simulink model "QuadCopter_3"  (R2018a)
settings: Solver=VariableStepAuto  StartTime=0.0  StopTime=t  RelTol=1e-3
values from neighbouring files (symbols this model uses):
  d = 2.4*10^-3    (= 0.0024)    [ScrValBackup.m]
  dx0 = 0    [ScrValBackup.m]
  dy0 = 0    [ScrValBackup.m]
  dz0 = 0    [ScrValBackup.m]
  g = 9.81    [ScrValBackup.m]
  Ixx = 5.9*10^-3    (= 0.0059)    [ScrValBackup.m]
  Iyy = 5.9*10^-3    (= 0.0059)    [ScrValBackup.m]
  Izz = 1.16*10^-3    (= 0.00116)    [ScrValBackup.m]
  kr = 0.1    [ScrValBackup.m]
  kt = 0.1    [ScrValBackup.m]
  l = 0.255    [ScrValBackup.m]
  m = 0.5    [ScrValBackup.m]
  p0 = 0.01    [ScrValBackup.m]
  phi0 = 5e-4    (= 0.0005)    [ScrValBackup.m]
  psi0 = 0    [ScrValBackup.m]
  q0 = -0.01    [ScrValBackup.m]
  r0 = 0.1177    [ScrValBackup.m]
  theta0 = -3e-4    (= -0.0003)    [ScrValBackup.m]
  x0 = 2    [ScrValBackup.m]
  x_coeff = A^-1*x_constr    [ScrValBackup.m]
  y0 = 3    [ScrValBackup.m]
  y_coeff = A^-1*y_constr    [ScrValBackup.m]
  z0 = 5    [ScrValBackup.m]
  z_coeff = A^-1*z_constr    [ScrValBackup.m]
libraries: simulink x5, aerolibutil x2
settings Model: Creator=giuseppe  LastModifiedBy=giuseppe
settings SolverCC: ZeroCrossAlgorithm=Adaptive
settings DebuggingCC: MaxConsecutiveZCsMsg=none

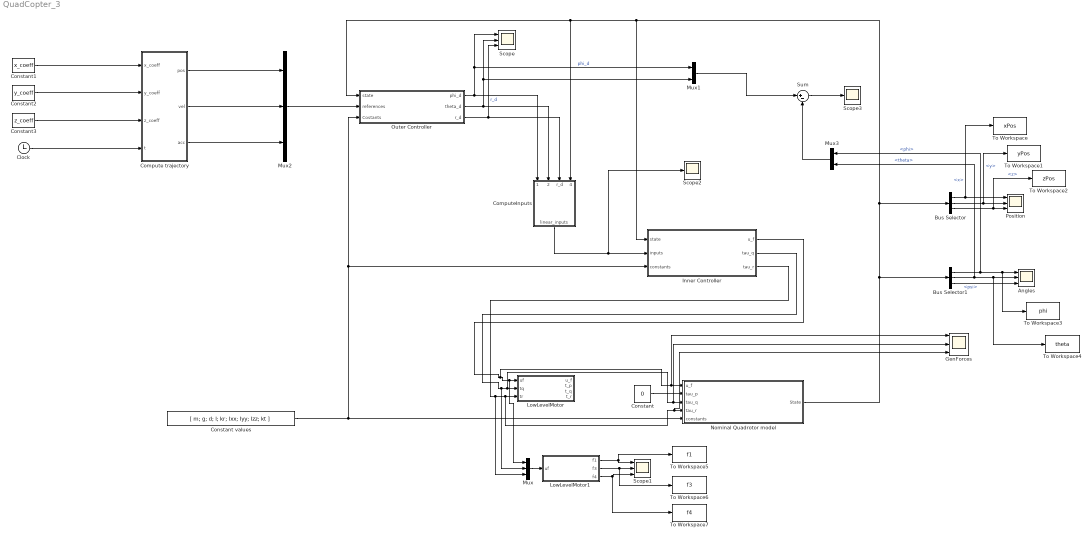
== system QuadCopter_3 ==
  Angles : Scope  NumInputPorts=3
  Bus Selector : BusSelector  OutputSignals=x,y,z
  Bus Selector1 : BusSelector  OutputSignals=phi,theta,psi
  Clock : Clock
  Compute trajectory : MATLAB Function  TreatAsAtomicUnit=on
  "ComputeInputs " : Subsystem
  Constant : Constant  Value=0
  Constant values : Constant  Value=[ m; g; d; l; kr; Ixx; Iyy; Izz; kt ]
  Constant1 : Constant  Value=x_coeff
  Constant2 : Constant  Value=y_coeff
  Constant3 : Constant  Value=z_coeff
  GenForces : Scope  NumInputPorts=3
  "Inner Controller " : Subsystem
  LowLevelMotor : Subsystem
  LowLevelMotor1 : Subsystem
  Mux : Mux  Inputs=3
  Mux1 : Mux  Inputs=2
  Mux2 : Mux  Inputs=3
  Mux3 : Mux  Inputs=2
  Nominal Quadrotor model : Subsystem
  "Outer Controller " : Subsystem
  Position : Scope  NumInputPorts=3
  Scope : Scope  NumInputPorts=3
  Scope1 : Scope  NumInputPorts=3
  Scope2 : Scope
  Scope3 : Scope
  Sum : Sum  Inputs=|+-
  To Workspace : ToWorkspace  VariableName=xPos  SaveFormat=Timeseries  SampleTime=-1
  To Workspace1 : ToWorkspace  VariableName=yPos  SaveFormat=Timeseries  SampleTime=-1
  To Workspace2 : ToWorkspace  VariableName=zPos  SaveFormat=Timeseries  SampleTime=-1
  To Workspace3 : ToWorkspace  VariableName=phi  SaveFormat=Timeseries  SampleTime=-1
  To Workspace4 : ToWorkspace  VariableName=theta  SaveFormat=Timeseries  SampleTime=-1
  To Workspace5 : ToWorkspace  VariableName=f1  SaveFormat=Timeseries  SampleTime=-1
  To Workspace6 : ToWorkspace  VariableName=f3  SaveFormat=Timeseries  SampleTime=-1
  To Workspace7 : ToWorkspace  VariableName=f4  SaveFormat=Timeseries  SampleTime=-1
  wires:
  Nominal Quadrotor model/1(State) -> "Inner Controller "/1(state), "ComputeInputs "/4(state), "Outer Controller "/1("state "), Bus Selector/1, Bus Selector1/1
  "Inner Controller "/3(tau_r) -> Mux/3, GenForces/3, Nominal Quadrotor model/4(tau_r), LowLevelMotor/3(tr)
  Constant values/1 -> "Outer Controller "/3(Costants), "Inner Controller "/3(constants), Nominal Quadrotor model/5(constants)
  "Outer Controller "/2(theta_d) -> "ComputeInputs "/2(theta_d), Mux1/2, Scope/2
  Constant3/1 -> Compute trajectory/3(z_coeff)
  "Outer Controller "/3(r_d) -> "ComputeInputs "/3(r_d), Scope/3  "r_d"
  "ComputeInputs "/1(linear_inputs) -> Scope2/1, "Inner Controller "/2(inputs)
  Constant1/1 -> Compute trajectory/1(x_coeff)
  Constant2/1 -> Compute trajectory/2(y_coeff)
  "Inner Controller "/1(u_f) -> GenForces/1, Nominal Quadrotor model/1(u_f), Mux/1, LowLevelMotor/1(uf)
  Clock/1 -> Compute trajectory/4(t)
  "Outer Controller "/1("phi_d ") -> "ComputeInputs "/1(phi_d), Mux1/1, Scope/1  "phi_d"
  Compute trajectory/3(acc) -> Mux2/3
  Compute trajectory/2(vel) -> Mux2/2
  Compute trajectory/1(pos) -> Mux2/1
  Mux2/1 -> "Outer Controller "/2(references)
  Bus Selector/1 -> To Workspace/1, Position/1  "<x>"
  Bus Selector/2 -> To Workspace1/1, Position/2  "<y>"
  Bus Selector/3 -> To Workspace2/1, Position/3  "<z>"
  Bus Selector1/1 -> Mux3/1, To Workspace3/1, Angles/1  "<phi>"
  Bus Selector1/2 -> Mux3/2, To Workspace4/1, Angles/2  "<theta>"
  Bus Selector1/3 -> Angles/3  "<psi>"
  Mux/1 -> LowLevelMotor1/1(uf)
  LowLevelMotor1/1(f1) -> Scope1/1, To Workspace5/1
  LowLevelMotor1/2(f3) -> To Workspace6/1, Scope1/2
  LowLevelMotor1/3(f4) -> To Workspace7/1, Scope1/3
  Constant/1 -> Nominal Quadrotor model/2(tau_p)
  "Inner Controller "/2(tau_q) -> Mux/2, GenForces/2, Nominal Quadrotor model/3(tau_q), LowLevelMotor/2("tq ")
  Mux3/1 -> Sum/2
  Mux1/1 -> Sum/1
  Sum/1 -> Scope3/1

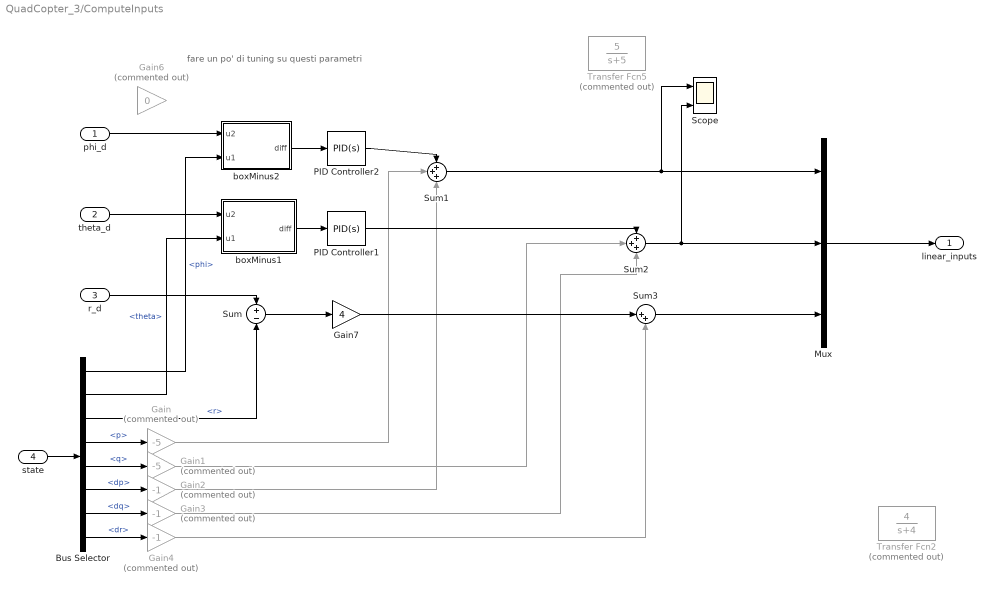
== system QuadCopter_3/ComputeInputs  ==
  note: fare un po' di tuning su questi parametri
  phi_d : Inport
  theta_d : Inport  Port=2
  r_d : Inport  Port=3
  state : Inport  Port=4
  Bus Selector : BusSelector  OutputSignals=phi,theta,r,p,q,dp,dq,dr
  Gain : Gain  Commented=on  Gain=-5
  Gain1 : Gain  Commented=on  Gain=-5
  Gain2 : Gain  Commented=on  Gain=-1
  Gain3 : Gain  Commented=on  Gain=-1
  Gain4 : Gain  Commented=on  Gain=-1
  Gain6 : Gain  Commented=on  Gain=0
  Gain7 : Gain  Gain=4
  Mux : Mux  Inputs=3
  PID Controller1 : simulink/Continuous/PID Controller  Controller=PID  TimeDomain=Continuous-time  SampleTime=-1  IntegratorMethod=Forward Euler  FilterMethod=Forward Euler  Form=Parallel  UseFilter=on  ControllerParametersSource=internal  P=100  I=10  D=30  N=100  InitialConditionSource=internal  InitialConditionForIntegrator=0  InitialConditionForFilter=0  ExternalReset=none  LimitOutput=off  UpperSaturationLimit=inf  LowerSaturationLimit=-inf  LinearizeAsGain=on  AntiWindupMode=none  Kb=1  TrackingMode=off  Kt=1  PParamMin=[]  PParamMax=[]  IParamMin=[]  IParamMax=[]  DParamMin=[]  DParamMax=[]  NParamMin=[]  NParamMax=[]  KbParamMin=[]  KbParamMax=[]  KtParamMin=[]  KtParamMax=[]  POutMin=[]  POutMax=[]  IOutMin=[]  IOutMax=[]  DOutMin=[]  DOutMax=[]  NOutMin=[]  NOutMax=[]  KbOutMin=[]  KbOutMax=[]  KtOutMin=[]  KtOutMax=[]  IntegratorOutMin=[]  IntegratorOutMax=[]  FilterOutMin=[]  FilterOutMax=[]  SumOutMin=[]  SumOutMax=[]  SumI1OutMin=[]  SumI1OutMax=[]  SumI2OutMin=[]  SumI2OutMax=[]  SumI3OutMin=[]  SumI3OutMax=[]  SumDOutMin=[]  SumDOutMax=[]  SaturationOutMin=[]  SaturationOutMax=[]  IntegratorContinuousStateAttributes=''  IntegratorStateMustResolveToSignalObject=off  IntegratorRTWStateStorageClass=Auto  FilterContinuousStateAttributes=''  FilterStateMustResolveToSignalObject=off  FilterRTWStateStorageClass=Auto  DifferentiatorICPrevScaledInput=0  DifferentiatorOutMin=[]  DifferentiatorOutMax=[]  FilterDiffOutCoefMin=[]  FilterDiffOutCoefMax=[]  SumDenOutMin=[]  SumDenOutMax=[]  SumNumOutMin=[]  SumNumOutMax=[]  ReciprocalOutMin=[]  ReciprocalOutMax=[]  DivideOutMin=[]  DivideOutMax=[]  TunerSelectOption=Transfer Function Based (PID Tuner App)
  PID Controller2 : simulink/Continuous/PID Controller  Controller=PID  TimeDomain=Continuous-time  SampleTime=-1  IntegratorMethod=Forward Euler  FilterMethod=Forward Euler  Form=Parallel  UseFilter=on  ControllerParametersSource=internal  P=100  I=10  D=30  N=100  InitialConditionSource=internal  InitialConditionForIntegrator=0  InitialConditionForFilter=0  ExternalReset=none  LimitOutput=off  UpperSaturationLimit=inf  LowerSaturationLimit=-inf  LinearizeAsGain=on  AntiWindupMode=none  Kb=1  TrackingMode=off  Kt=1  PParamMin=[]  PParamMax=[]  IParamMin=[]  IParamMax=[]  DParamMin=[]  DParamMax=[]  NParamMin=[]  NParamMax=[]  KbParamMin=[]  KbParamMax=[]  KtParamMin=[]  KtParamMax=[]  POutMin=[]  POutMax=[]  IOutMin=[]  IOutMax=[]  DOutMin=[]  DOutMax=[]  NOutMin=[]  NOutMax=[]  KbOutMin=[]  KbOutMax=[]  KtOutMin=[]  KtOutMax=[]  IntegratorOutMin=[]  IntegratorOutMax=[]  FilterOutMin=[]  FilterOutMax=[]  SumOutMin=[]  SumOutMax=[]  SumI1OutMin=[]  SumI1OutMax=[]  SumI2OutMin=[]  SumI2OutMax=[]  SumI3OutMin=[]  SumI3OutMax=[]  SumDOutMin=[]  SumDOutMax=[]  SaturationOutMin=[]  SaturationOutMax=[]  IntegratorContinuousStateAttributes=''  IntegratorStateMustResolveToSignalObject=off  IntegratorRTWStateStorageClass=Auto  FilterContinuousStateAttributes=''  FilterStateMustResolveToSignalObject=off  FilterRTWStateStorageClass=Auto  DifferentiatorICPrevScaledInput=0  DifferentiatorOutMin=[]  DifferentiatorOutMax=[]  FilterDiffOutCoefMin=[]  FilterDiffOutCoefMax=[]  SumDenOutMin=[]  SumDenOutMax=[]  SumNumOutMin=[]  SumNumOutMax=[]  ReciprocalOutMin=[]  ReciprocalOutMax=[]  DivideOutMin=[]  DivideOutMax=[]  TunerSelectOption=Transfer Function Based (PID Tuner App)
  Scope : Scope  NumInputPorts=2
  Sum : Sum  Inputs=+-
  Sum1 : Sum  Inputs=+++
  Sum2 : Sum  Inputs=+++
  Sum3 : Sum  Inputs=|++
  Transfer Fcn2 : TransferFcn  Commented=on  Numerator=[4]  Denominator=[1 4]
  Transfer Fcn5 : TransferFcn  Commented=on  Numerator=[5]  Denominator=[1 5]
  boxMinus1 : MATLAB Function  TreatAsAtomicUnit=on
  boxMinus2 : MATLAB Function  TreatAsAtomicUnit=on
  linear_inputs : Outport
  wires:
  r_d/1 -> Sum/1
  state/1 -> Bus Selector/1
  Bus Selector/1 -> boxMinus2/2(u1)  "<phi>"
  Bus Selector/2 -> boxMinus1/2(u1)  "<theta>"
  Bus Selector/3 -> Sum/2  "<r>"
  Bus Selector/4 -> Gain/1  "<p>"
  Bus Selector/5 -> Gain1/1  "<q>"
  Bus Selector/6 -> Gain2/1  "<dp>"
  Bus Selector/7 -> Gain3/1  "<dq>"
  Bus Selector/8 -> Gain4/1  "<dr>"
  boxMinus2/1(diff) -> PID Controller2/1
  Gain/1 -> Sum1/2
  Gain2/1 -> Sum1/3
  boxMinus1/1(diff) -> PID Controller1/1
  Gain1/1 -> Sum2/2
  Gain3/1 -> Sum2/3
  Sum/1 -> Gain7/1
  Gain4/1 -> Sum3/2
  Sum3/1 -> Mux/3
  Mux/1 -> linear_inputs/1
  PID Controller1/1 -> Sum2/1
  Gain7/1 -> Sum3/1
  phi_d/1 -> boxMinus2/1(u2)
  theta_d/1 -> boxMinus1/1(u2)
  PID Controller2/1 -> Sum1/1
  Sum1/1 -> Scope/1, Mux/1
  Sum2/1 -> Scope/2, Mux/2

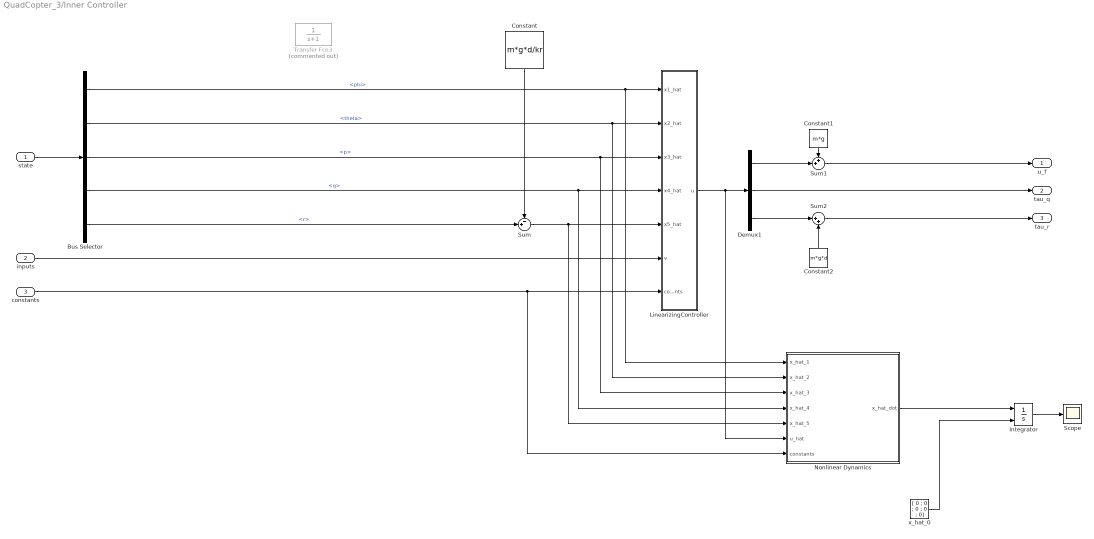
== system QuadCopter_3/Inner Controller  ==
  state : Inport
  inputs : Inport  Port=2
  constants : Inport  Port=3
  Bus Selector : BusSelector  OutputSignals=phi,theta,p,q,r
  Constant : Constant  Value=m*g*d/kr
  Constant1 : Constant  Value=m*g
  Constant2 : Constant  Value=m*g*d
  Demux1 : Demux  Outputs=3
  Integrator : Integrator  InitialConditionSource=external
  LinearizingController : MATLAB Function  TreatAsAtomicUnit=on
  "Nonlinear Dynamics " : MATLAB Function  TreatAsAtomicUnit=on
  Scope : Scope
  Sum : Sum  Inputs=-+|
  Sum1 : Sum  Inputs=++|
  Sum2 : Sum  Inputs=|++
  Transfer Fcn3 : TransferFcn  Commented=on  Denominator=[1 1]
  x_hat_0 : Constant  Value=[ 0 ; 0 ; 0 ; 0 ; 0]
  u_f : Outport
  tau_q : Outport  Port=2
  tau_r : Outport  Port=3
  wires:
  Bus Selector/3 -> "Nonlinear Dynamics "/3(x_hat_3), LinearizingController/3(x3_hat)  "<p>"
  Bus Selector/4 -> "Nonlinear Dynamics "/4(x_hat_4), LinearizingController/4(x4_hat)  "<q>"
  "Nonlinear Dynamics "/1(x_hat_dot) -> Integrator/1
  x_hat_0/1 -> Integrator/2
  Constant/1 -> Sum/1
  Sum/1 -> LinearizingController/5(x5_hat), "Nonlinear Dynamics "/5(x_hat_5)
  Demux1/3 -> Sum2/1
  Demux1/1 -> Sum1/2
  Constant1/1 -> Sum1/1
  Sum1/1 -> u_f/1
  Demux1/2 -> tau_q/1
  Constant2/1 -> Sum2/2
  Sum2/1 -> tau_r/1
  LinearizingController/1(u) -> "Nonlinear Dynamics "/6(u_hat), Demux1/1
  Integrator/1 -> Scope/1
  constants/1 -> "Nonlinear Dynamics "/7(constants), LinearizingController/7(constants)
  Bus Selector/5 -> Sum/2  "<r>"
  Bus Selector/1 -> "Nonlinear Dynamics "/1(x_hat_1), LinearizingController/1(x1_hat)  "<phi>"
  Bus Selector/2 -> "Nonlinear Dynamics "/2(x_hat_2), LinearizingController/2(x2_hat)  "<theta>"
  inputs/1 -> LinearizingController/6(v)
  state/1 -> Bus Selector/1

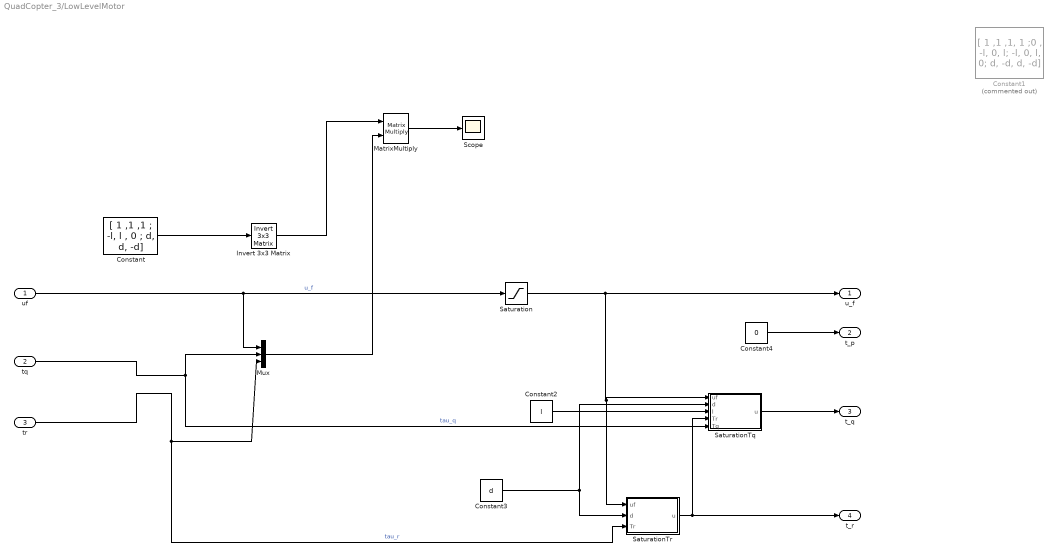
== system QuadCopter_3/LowLevelMotor ==
  uf : Inport
  "tq " : Inport  Port=2
  tr : Inport  Port=3
  Constant : Constant  Value=[ 1 ,1 ,1 ; -l, l , 0 ; d, d, -d]
  Constant1 : Constant  Commented=on  Value="[ 1 ,1 ,1, 1 ;0 , -l, 0, l;  -l, 0, l, 0; d, -d, d, -d]"
  Constant2 : Constant  Value=l
  Constant3 : Constant  Value=d
  Constant4 : Constant  Value=0
  Invert 3x3 Matrix : aerolibutil/Invert  3x3 Matrix
  MatrixMultiply : Product  Multiplication=Matrix(*)
  Mux : Mux  Inputs=3
  Saturation : Saturate  UpperLimit=15
  SaturationTq : MATLAB Function  TreatAsAtomicUnit=on
  SaturationTr : MATLAB Function  TreatAsAtomicUnit=on
  Scope : Scope
  u_f : Outport
  t_p : Outport  Port=2
  t_q : Outport  Port=3
  t_r : Outport  Port=4
  wires:
  "tq "/1 -> SaturationTq/5(Tq), Mux/2  "tau_q"
  tr/1 -> Mux/3, SaturationTr/3(Tr)  "tau_r"
  uf/1 -> Mux/1, Saturation/1  "u_f"
  Constant/1 -> Invert 3x3 Matrix/1
  Constant4/1 -> t_p/1
  Constant3/1 -> SaturationTq/2(d), SaturationTr/2(d)
  SaturationTr/1(u) -> SaturationTq/4(Tr), t_r/1
  SaturationTq/1(u) -> t_q/1
  Invert 3x3 Matrix/1 -> MatrixMultiply/1
  Saturation/1 -> SaturationTr/1(uf), SaturationTq/1(uf), u_f/1
  Mux/1 -> MatrixMultiply/2
  MatrixMultiply/1 -> Scope/1
  Constant2/1 -> SaturationTq/3(l)

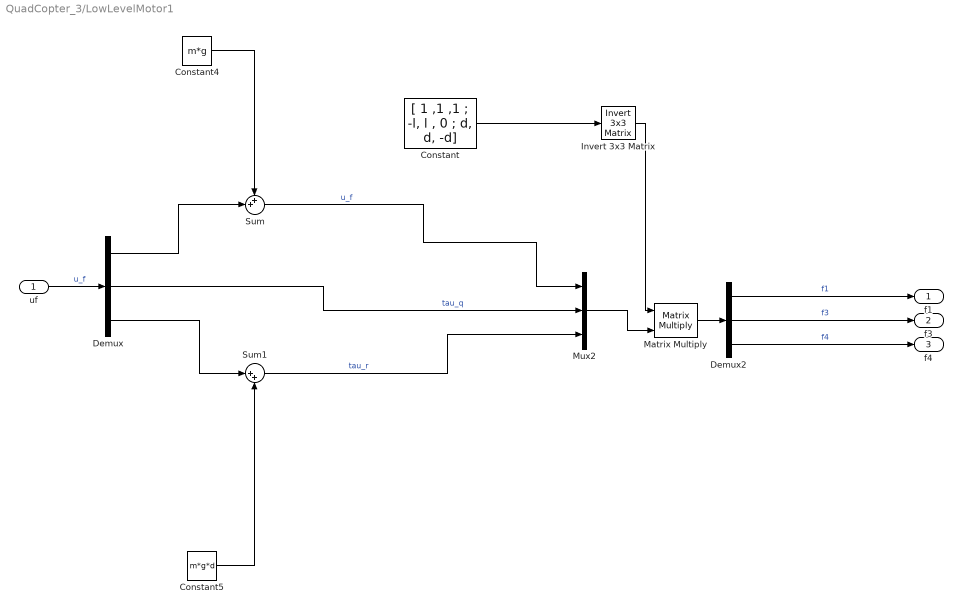
== system QuadCopter_3/LowLevelMotor1 ==
  uf : Inport
  Constant : Constant  Value=[ 1 ,1 ,1 ; -l, l , 0 ; d, d, -d]
  Constant4 : Constant  Value=m*g
  Constant5 : Constant  Value=m*g*d
  Demux : Demux  Outputs=3
  Demux2 : Demux  Outputs=3
  Invert 3x3 Matrix : aerolibutil/Invert  3x3 Matrix
  Matrix Multiply : Product  Multiplication=Matrix(*)
  Mux2 : Mux  Inputs=3
  Sum : Sum  Inputs=++|
  Sum1 : Sum  Inputs=|++
  f1 : Outport
  f3 : Outport  Port=2
  f4 : Outport  Port=3
  wires:
  Demux/2 -> Mux2/2  "tau_q"
  Invert 3x3 Matrix/1 -> Matrix Multiply/1
  Sum1/1 -> Mux2/3  "tau_r"
  Mux2/1 -> Matrix Multiply/2
  Matrix Multiply/1 -> Demux2/1
  Sum/1 -> Mux2/1  "u_f"
  Constant/1 -> Invert 3x3 Matrix/1
  uf/1 -> Demux/1  "u_f"
  Constant4/1 -> Sum/1
  Demux/1 -> Sum/2
  Demux/3 -> Sum1/1
  Constant5/1 -> Sum1/2
  Demux2/1 -> f1/1  "f1"
  Demux2/2 -> f3/1  "f3"
  Demux2/3 -> f4/1  "f4"

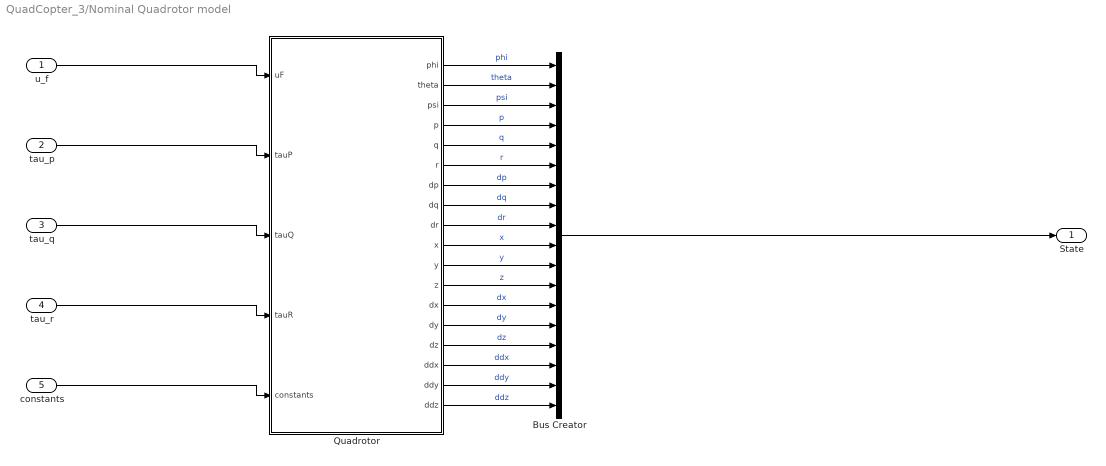
== system QuadCopter_3/Nominal Quadrotor model ==
  u_f : Inport
  tau_p : Inport  Port=2
  tau_q : Inport  Port=3
  tau_r : Inport  Port=4
  constants : Inport  Port=5
  Bus Creator : BusCreator  Inputs=18
  "Quadrotor " : Subsystem
  State : Outport
  wires:
  u_f/1 -> "Quadrotor "/1(uF)
  tau_q/1 -> "Quadrotor "/3(tauQ)
  tau_r/1 -> "Quadrotor "/4(tauR)
  constants/1 -> "Quadrotor "/5(constants)
  tau_p/1 -> "Quadrotor "/2(tauP)
  Bus Creator/1 -> State/1
  "Quadrotor "/1(phi) -> Bus Creator/1  "phi"
  "Quadrotor "/2(theta) -> Bus Creator/2  "theta"
  "Quadrotor "/3(psi) -> Bus Creator/3  "psi"
  "Quadrotor "/4(p) -> Bus Creator/4  "p"
  "Quadrotor "/5(q) -> Bus Creator/5  "q"
  "Quadrotor "/6(r) -> Bus Creator/6  "r"
  "Quadrotor "/7(dp) -> Bus Creator/7  "dp"
  "Quadrotor "/8(dq) -> Bus Creator/8  "dq"
  "Quadrotor "/9(dr) -> Bus Creator/9  "dr"
  "Quadrotor "/10(x) -> Bus Creator/10  "x"
  "Quadrotor "/11(y) -> Bus Creator/11  "y"
  "Quadrotor "/12(z) -> Bus Creator/12  "z"
  "Quadrotor "/13(dx) -> Bus Creator/13  "dx"
  "Quadrotor "/14(dy) -> Bus Creator/14  "dy"
  "Quadrotor "/15(dz) -> Bus Creator/15  "dz"
  "Quadrotor "/16(ddx) -> Bus Creator/16  "ddx"
  "Quadrotor "/17(ddy) -> Bus Creator/17  "ddy"
  "Quadrotor "/18(ddz) -> Bus Creator/18  "ddz"

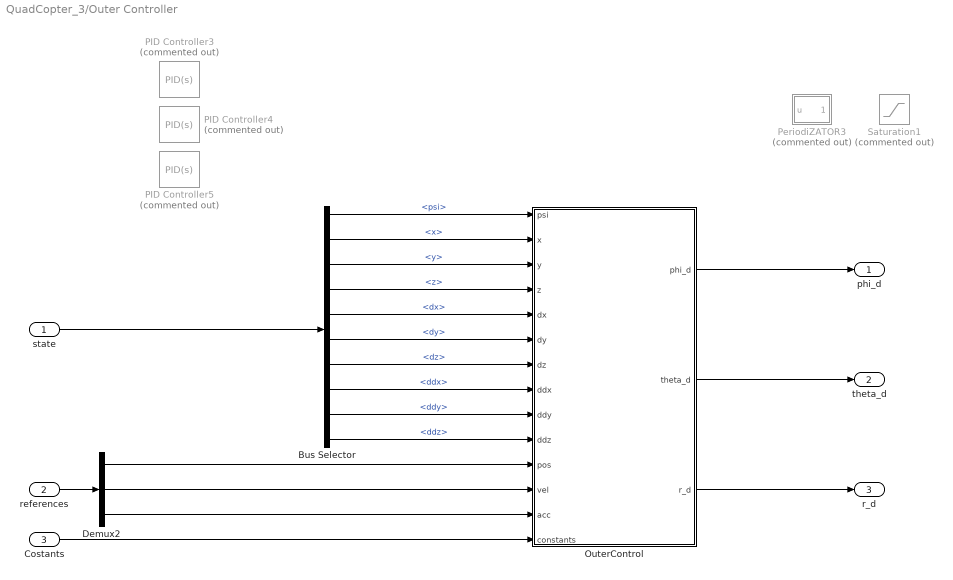
== system QuadCopter_3/Outer Controller  ==
  "state " : Inport  SampleTime=0.1
  references : Inport  Port=2
  Costants : Inport  Port=3
  Bus Selector : BusSelector  OutputSignals=psi,x,y,z,dx,dy,dz,ddx,ddy,ddz
  Demux2 : Demux  Outputs=3
  OuterControl : MATLAB Function  TreatAsAtomicUnit=on
  PID Controller3 : simulink/Continuous/PID Controller  Commented=on  Controller=PID  TimeDomain=Continuous-time  SampleTime=-1  IntegratorMethod=Forward Euler  FilterMethod=Forward Euler  Form=Parallel  UseFilter=on  ControllerParametersSource=internal  P=-3.31812549008861e-05  I=-2.04327645124417e-11  D=-11.9723513961423  N=0.0120629646409386  InitialConditionSource=internal  InitialConditionForIntegrator=0  InitialConditionForFilter=0  ExternalReset=none  LimitOutput=off  UpperSaturationLimit=inf  LowerSaturationLimit=-inf  LinearizeAsGain=on  AntiWindupMode=none  Kb=1  TrackingMode=off  Kt=1  PParamMin=[]  PParamMax=[]  IParamMin=[]  IParamMax=[]  DParamMin=[]  DParamMax=[]  NParamMin=[]  NParamMax=[]  KbParamMin=[]  KbParamMax=[]  KtParamMin=[]  KtParamMax=[]  POutMin=[]  POutMax=[]  IOutMin=[]  IOutMax=[]  DOutMin=[]  DOutMax=[]  NOutMin=[]  NOutMax=[]  KbOutMin=[]  KbOutMax=[]  KtOutMin=[]  KtOutMax=[]  IntegratorOutMin=[]  IntegratorOutMax=[]  FilterOutMin=[]  FilterOutMax=[]  SumOutMin=[]  SumOutMax=[]  SumI1OutMin=[]  SumI1OutMax=[]  SumI2OutMin=[]  SumI2OutMax=[]  SumI3OutMin=[]  SumI3OutMax=[]  SumDOutMin=[]  SumDOutMax=[]  SaturationOutMin=[]  SaturationOutMax=[]  IntegratorContinuousStateAttributes=''  IntegratorStateMustResolveToSignalObject=off  IntegratorRTWStateStorageClass=Auto  FilterContinuousStateAttributes=''  FilterStateMustResolveToSignalObject=off  FilterRTWStateStorageClass=Auto  DifferentiatorICPrevScaledInput=0  DifferentiatorOutMin=[]  DifferentiatorOutMax=[]  FilterDiffOutCoefMin=[]  FilterDiffOutCoefMax=[]  SumDenOutMin=[]  SumDenOutMax=[]  SumNumOutMin=[]  SumNumOutMax=[]  ReciprocalOutMin=[]  ReciprocalOutMax=[]  DivideOutMin=[]  DivideOutMax=[]  TunerSelectOption=Transfer Function Based (PID Tuner App)
  PID Controller4 : simulink/Continuous/PID Controller  Commented=on  Controller=PID  TimeDomain=Continuous-time  SampleTime=-1  IntegratorMethod=Forward Euler  FilterMethod=Forward Euler  Form=Parallel  UseFilter=on  ControllerParametersSource=internal  P=-3.31812549008861e-05  I=-2.04327645124417e-11  D=-11.9723513961423  N=0.0120629646409386  InitialConditionSource=internal  InitialConditionForIntegrator=0  InitialConditionForFilter=0  ExternalReset=none  LimitOutput=off  UpperSaturationLimit=inf  LowerSaturationLimit=-inf  LinearizeAsGain=on  AntiWindupMode=none  Kb=1  TrackingMode=off  Kt=1  PParamMin=[]  PParamMax=[]  IParamMin=[]  IParamMax=[]  DParamMin=[]  DParamMax=[]  NParamMin=[]  NParamMax=[]  KbParamMin=[]  KbParamMax=[]  KtParamMin=[]  KtParamMax=[]  POutMin=[]  POutMax=[]  IOutMin=[]  IOutMax=[]  DOutMin=[]  DOutMax=[]  NOutMin=[]  NOutMax=[]  KbOutMin=[]  KbOutMax=[]  KtOutMin=[]  KtOutMax=[]  IntegratorOutMin=[]  IntegratorOutMax=[]  FilterOutMin=[]  FilterOutMax=[]  SumOutMin=[]  SumOutMax=[]  SumI1OutMin=[]  SumI1OutMax=[]  SumI2OutMin=[]  SumI2OutMax=[]  SumI3OutMin=[]  SumI3OutMax=[]  SumDOutMin=[]  SumDOutMax=[]  SaturationOutMin=[]  SaturationOutMax=[]  IntegratorContinuousStateAttributes=''  IntegratorStateMustResolveToSignalObject=off  IntegratorRTWStateStorageClass=Auto  FilterContinuousStateAttributes=''  FilterStateMustResolveToSignalObject=off  FilterRTWStateStorageClass=Auto  DifferentiatorICPrevScaledInput=0  DifferentiatorOutMin=[]  DifferentiatorOutMax=[]  FilterDiffOutCoefMin=[]  FilterDiffOutCoefMax=[]  SumDenOutMin=[]  SumDenOutMax=[]  SumNumOutMin=[]  SumNumOutMax=[]  ReciprocalOutMin=[]  ReciprocalOutMax=[]  DivideOutMin=[]  DivideOutMax=[]  TunerSelectOption=Transfer Function Based (PID Tuner App)
  PID Controller5 : simulink/Continuous/PID Controller  Commented=on  Controller=PID  TimeDomain=Continuous-time  SampleTime=-1  IntegratorMethod=Forward Euler  FilterMethod=Forward Euler  Form=Parallel  UseFilter=on  ControllerParametersSource=internal  P=-3.31812549008861e-05  I=-2.04327645124417e-11  D=-11.9723513961423  N=0.0120629646409386  InitialConditionSource=internal  InitialConditionForIntegrator=0  InitialConditionForFilter=0  ExternalReset=none  LimitOutput=off  UpperSaturationLimit=inf  LowerSaturationLimit=-inf  LinearizeAsGain=on  AntiWindupMode=none  Kb=1  TrackingMode=off  Kt=1  PParamMin=[]  PParamMax=[]  IParamMin=[]  IParamMax=[]  DParamMin=[]  DParamMax=[]  NParamMin=[]  NParamMax=[]  KbParamMin=[]  KbParamMax=[]  KtParamMin=[]  KtParamMax=[]  POutMin=[]  POutMax=[]  IOutMin=[]  IOutMax=[]  DOutMin=[]  DOutMax=[]  NOutMin=[]  NOutMax=[]  KbOutMin=[]  KbOutMax=[]  KtOutMin=[]  KtOutMax=[]  IntegratorOutMin=[]  IntegratorOutMax=[]  FilterOutMin=[]  FilterOutMax=[]  SumOutMin=[]  SumOutMax=[]  SumI1OutMin=[]  SumI1OutMax=[]  SumI2OutMin=[]  SumI2OutMax=[]  SumI3OutMin=[]  SumI3OutMax=[]  SumDOutMin=[]  SumDOutMax=[]  SaturationOutMin=[]  SaturationOutMax=[]  IntegratorContinuousStateAttributes=''  IntegratorStateMustResolveToSignalObject=off  IntegratorRTWStateStorageClass=Auto  FilterContinuousStateAttributes=''  FilterStateMustResolveToSignalObject=off  FilterRTWStateStorageClass=Auto  DifferentiatorICPrevScaledInput=0  DifferentiatorOutMin=[]  DifferentiatorOutMax=[]  FilterDiffOutCoefMin=[]  FilterDiffOutCoefMax=[]  SumDenOutMin=[]  SumDenOutMax=[]  SumNumOutMin=[]  SumNumOutMax=[]  ReciprocalOutMin=[]  ReciprocalOutMax=[]  DivideOutMin=[]  DivideOutMax=[]  TunerSelectOption=Transfer Function Based (PID Tuner App)
  PeriodiZATOR3 : MATLAB Function  Commented=on  TreatAsAtomicUnit=on
  Saturation1 : Saturate  Commented=on  UpperLimit=5  LowerLimit=0
  "phi_d " : Outport
  theta_d : Outport  Port=2
  r_d : Outport  Port=3
  wires:
  Costants/1 -> OuterControl/14(constants)
  references/1 -> Demux2/1
  OuterControl/3(r_d) -> r_d/1
  OuterControl/1(phi_d) -> "phi_d "/1
  OuterControl/2(theta_d) -> theta_d/1
  "state "/1 -> Bus Selector/1
  Bus Selector/10 -> OuterControl/10(ddz)  "<ddz>"
  Bus Selector/9 -> OuterControl/9(ddy)  "<ddy>"
  Bus Selector/8 -> OuterControl/8(ddx)  "<ddx>"
  Bus Selector/7 -> OuterControl/7(dz)  "<dz>"
  Bus Selector/6 -> OuterControl/6(dy)  "<dy>"
  Bus Selector/5 -> OuterControl/5(dx)  "<dx>"
  Bus Selector/4 -> OuterControl/4(z)  "<z>"
  Bus Selector/3 -> OuterControl/3(y)  "<y>"
  Bus Selector/2 -> OuterControl/2(x)  "<x>"
  Bus Selector/1 -> OuterControl/1(psi)  "<psi>"
  Demux2/1 -> OuterControl/11(pos)
  Demux2/2 -> OuterControl/12(vel)
  Demux2/3 -> OuterControl/13(acc)

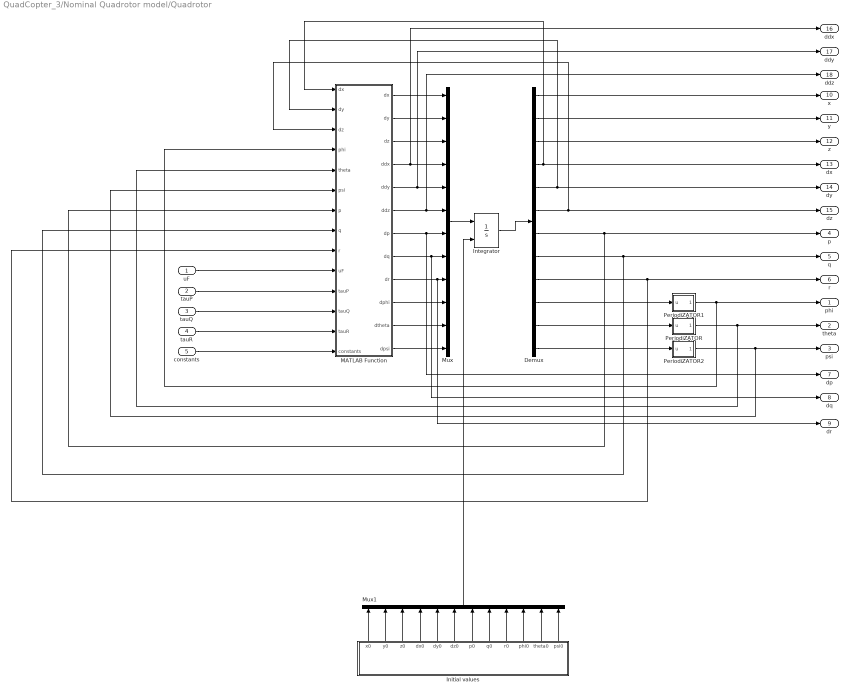
== system QuadCopter_3/Nominal Quadrotor model/Quadrotor  ==
  uF : Inport
  tauP : Inport  Port=2
  tauQ : Inport  Port=3
  tauR : Inport  Port=4
  constants : Inport  Port=5
  Demux : Demux  Outputs=12
  "Initial values " : Subsystem
  Integrator : Integrator  InitialConditionSource=external
  MATLAB Function : MATLAB Function  TreatAsAtomicUnit=on
  Mux : Mux  Inputs=12
  Mux1 : Mux  Inputs=12
  PeriodiZATOR : MATLAB Function  TreatAsAtomicUnit=on
  PeriodiZATOR1 : MATLAB Function  TreatAsAtomicUnit=on
  PeriodiZATOR2 : MATLAB Function  TreatAsAtomicUnit=on
  phi : Outport
  theta : Outport  Port=2
  psi : Outport  Port=3
  p : Outport  Port=4
  q : Outport  Port=5
  r : Outport  Port=6
  dp : Outport  Port=7
  dq : Outport  Port=8
  dr : Outport  Port=9
  x : Outport  Port=10
  y : Outport  Port=11
  z : Outport  Port=12
  dx : Outport  Port=13
  dy : Outport  Port=14
  dz : Outport  Port=15
  ddx : Outport  Port=16
  ddy : Outport  Port=17
  ddz : Outport  Port=18
  wires:
  uF/1 -> MATLAB Function/10(uF)
  tauP/1 -> MATLAB Function/11(tauP)
  tauQ/1 -> MATLAB Function/12(tauQ)
  tauR/1 -> MATLAB Function/13(tauR)
  PeriodiZATOR/1(angle) -> MATLAB Function/5(theta), theta/1
  PeriodiZATOR1/1(angle) -> MATLAB Function/4(phi), phi/1
  PeriodiZATOR2/1(angle) -> MATLAB Function/6(psi), psi/1
  constants/1 -> MATLAB Function/14(constants)
  MATLAB Function/1(dx) -> Mux/1
  MATLAB Function/2(dy) -> Mux/2
  MATLAB Function/3(dz) -> Mux/3
  MATLAB Function/4(ddx) -> ddx/1, Mux/4
  MATLAB Function/5(ddy) -> ddy/1, Mux/5
  MATLAB Function/6(ddz) -> Mux/6, ddz/1
  MATLAB Function/10(dphi) -> Mux/10
  MATLAB Function/11(dtheta) -> Mux/11
  MATLAB Function/12(dpsi) -> Mux/12
  Mux/1 -> Integrator/1
  "Initial values "/1(x0) -> Mux1/1
  "Initial values "/2(y0) -> Mux1/2
  "Initial values "/3(z0) -> Mux1/3
  "Initial values "/4(dx0) -> Mux1/4
  "Initial values "/5(dy0) -> Mux1/5
  "Initial values "/6(dz0) -> Mux1/6
  "Initial values "/7(p0) -> Mux1/7
  "Initial values "/8(q0) -> Mux1/8
  "Initial values "/9(r0) -> Mux1/9
  "Initial values "/10(phi0) -> Mux1/10
  "Initial values "/11(theta0) -> Mux1/11
  "Initial values "/12(psi0) -> Mux1/12
  Mux1/1 -> Integrator/2
  Integrator/1 -> Demux/1
  Demux/1 -> x/1
  Demux/2 -> y/1
  Demux/3 -> z/1
  Demux/5 -> dy/1, MATLAB Function/2("dy ")
  Demux/6 -> dz/1, MATLAB Function/3("dz ")
  Demux/10 -> PeriodiZATOR1/1(u)
  Demux/11 -> PeriodiZATOR/1(u)
  Demux/12 -> PeriodiZATOR2/1(u)
  Demux/9 -> MATLAB Function/9(r), r/1
  MATLAB Function/7(dp) -> Mux/7, dp/1
  MATLAB Function/8(dq) -> Mux/8, dq/1
  Demux/7 -> MATLAB Function/7(p), p/1
  Demux/8 -> MATLAB Function/8(q), q/1
  MATLAB Function/9(dr) -> dr/1, Mux/9
  Demux/4 -> dx/1, MATLAB Function/1("dx ")

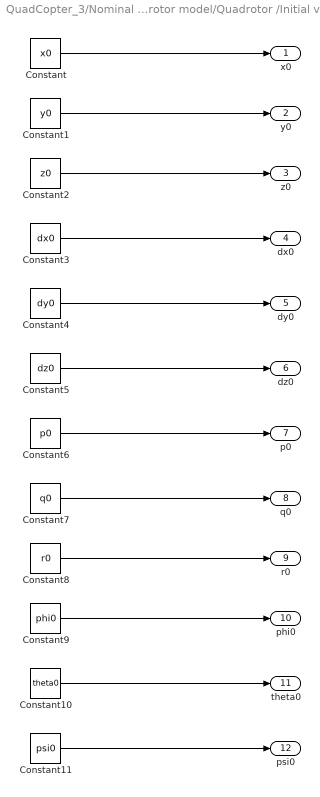
== system QuadCopter_3/Nominal Quadrotor model/Quadrotor /Initial values  ==
  Constant : Constant  Value=x0
  Constant1 : Constant  Value=y0
  Constant10 : Constant  Value=theta0
  Constant11 : Constant  Value=psi0
  Constant2 : Constant  Value=z0
  Constant3 : Constant  Value=dx0
  Constant4 : Constant  Value=dy0
  Constant5 : Constant  Value=dz0
  Constant6 : Constant  Value=p0
  Constant7 : Constant  Value=q0
  Constant8 : Constant  Value=r0
  Constant9 : Constant  Value=phi0
  x0 : Outport
  y0 : Outport  Port=2
  z0 : Outport  Port=3
  dx0 : Outport  Port=4
  dy0 : Outport  Port=5
  dz0 : Outport  Port=6
  p0 : Outport  Port=7
  q0 : Outport  Port=8
  r0 : Outport  Port=9
  phi0 : Outport  Port=10
  theta0 : Outport  Port=11
  psi0 : Outport  Port=12
  wires:
  Constant/1 -> x0/1
  Constant1/1 -> y0/1
  Constant2/1 -> z0/1
  Constant3/1 -> dx0/1
  Constant4/1 -> dy0/1
  Constant5/1 -> dz0/1
  Constant6/1 -> p0/1
  Constant7/1 -> q0/1
  Constant8/1 -> r0/1
  Constant9/1 -> phi0/1
  Constant10/1 -> theta0/1
  Constant11/1 -> psi0/1

== matlab function QuadCopter_3/Inner Controller /LinearizingController ==
  data: x1_hat input; u output; x2_hat input; x3_hat input; x4_hat input; x5_hat input; v input; constants input
function u = fcn(x1_hat,x2_hat,x3_hat,x4_hat,x5_hat, v, constants)

m= constants(1,1);
g= constants(2,1);
d= constants(3,1);
l= constants(4,1);
kr= constants(5,1);
Ixx= constants(6,1);
Iyy= constants(7,1);
Izz= constants(8,1);

alfa = zeros(3,1);

%% Non-robust feedback-linearation

alfa(1,1) = (2*Ixx*((kr*x3_hat - x4_hat*(x5_hat + (d*g*m)/kr)*(Ixx - Izz))/Ixx + (sin(x1_hat)*tan(x2_hat)*(x5_hat + (d*g*m)/kr) - x4_hat*cos(x1_hat)*tan(x2_hat))*(x3_hat + cos(x1_hat)*tan(x2_hat)*(x5_hat + (d*g*m)/kr) + x4_hat*sin(x1_hat)*tan(x2_hat)) + (sin(x1_hat)*(x5_hat + (d*g*m)/kr) - x4_hat*cos(x1_hat))*(cos(x1_hat)*(x5_hat + (d*g*m)/kr)*(tan(x2_hat)^2 + 1) + x4_hat*sin(x1_hat)*(tan(x2_hat)^2 + 1)) + (sin(x1_hat)*tan(x2_hat)*(kr*x4_hat + x3_hat*(x5_hat + (d*g*m)/kr)*(Ixx - Izz)))/Ixx + (kr*x5_hat*cos(x1_hat)*tan(x2_hat))/Izz))/l - (2*Ixx*sin(x1_hat)*tan(x2_hat)*((cos(x1_hat)*(x5_hat + (d*g*m)/kr) + x4_hat*sin(x1_hat))*(x3_hat + cos(x1_hat)*tan(x2_hat)*(x5_hat + (d*g*m)/kr) + x4_hat*sin(x1_hat)*tan(x2_hat)) + (cos(x1_hat)*(kr*x4_hat + x3_hat*(x5_hat + (d*g*m)/kr)*(Ixx - Izz)))/Ixx - (kr*x5_hat*sin(x1_hat))/Izz))/(l*cos(x1_hat)) - (kr*x5_hat*(2*Ixx*d*cos(x1_hat)^2*tan(x2_hat) - Izz*l*cos(x1_hat) + 2*Ixx*d*sin(x1_hat)^2*tan(x2_hat)))/(Izz*d*l*cos(x1_hat));
alfa(2,1) = (Ixx*((cos(x1_hat)*(x5_hat + (d*g*m)/kr) + x4_hat*sin(x1_hat))*(x3_hat + cos(x1_hat)*tan(x2_hat)*(x5_hat + (d*g*m)/kr) + x4_hat*sin(x1_hat)*tan(x2_hat)) + (cos(x1_hat)*(kr*x4_hat + x3_hat*(x5_hat + (d*g*m)/kr)*(Ixx - Izz)))/Ixx - (kr*x5_hat*sin(x1_hat))/Izz))/cos(x1_hat) + (Ixx*kr*x5_hat*sin(x1_hat))/(Izz*cos(x1_hat));
alfa(3,1) = kr*x5_hat;


beta =  [
         (2*Ixx)/l, -(2*Ixx*sin(x1_hat)*sin(x2_hat))/(l*cos(x1_hat)*cos(x2_hat)), -(2*Ixx*d*sin(x2_hat)-Izz*l*cos(x1_hat)*cos(x2_hat))/(d*l*cos(x1_hat)*cos(x2_hat));
         0,                                              Ixx/cos(x1_hat),                                                        (Ixx*sin(x1_hat))/cos(x1_hat);
         0,                                                            0,                                                                                  Izz];

%% Robust feedback linearization

% alfa(1,1) = x1_hat*((d*g*m*((2*Ixx*((d*g*m)/kr + (d*g*m*(Ixx - Izz))/(Ixx*kr)))/l + (2*kr*sin(x1_hat)*tan(x2_hat))/(l*cos(x1_hat))))/kr - (2*Ixx*d^2*g^2*m^2)/(kr^2*l)) - (sin(x1_hat)*(x5_hat + (d*g*m)/kr) - x4_hat*cos(x1_hat))*((2*Ixx*((d*g*m)/kr + (d*g*m*(Ixx - Izz))/(Ixx*kr)))/l + (2*kr*sin(x1_hat)*tan(x2_hat))/(l*cos(x1_hat))) + x2_hat*((d*g*m*((2*kr)/l - (2*Ixx*sin(x1_hat)*tan(x2_hat)*((d*g*m)/kr + (d*g*m*(Ixx - Izz))/(Ixx*kr)))/(l*cos(x1_hat))))/kr + (2*Ixx*d^2*g^2*m^2*sin(x1_hat)*tan(x2_hat))/(kr^2*l*cos(x1_hat))) - ((2*kr)/l - (2*Ixx*sin(x1_hat)*tan(x2_hat)*((d*g*m)/kr + (d*g*m*(Ixx - Izz))/(Ixx*kr)))/(l*cos(x1_hat)))*(x3_hat + cos(x1_hat)*tan(x2_hat)*(x5_hat + (d*g*m)/kr) + x4_hat*sin(x1_hat)*tan(x2_hat)) + (2*Ixx*((kr*x3_hat - x4_hat*(x5_hat + (d*g*m)/kr)*(Ixx - Izz))/Ixx + (sin(x1_hat)*tan(x2_hat)*(x5_hat + (d*g*m)/kr) - x4_hat*cos(x1_hat)*tan(x2_hat))*(x3_hat + cos(x1_hat)*tan(x2_hat)*(x5_hat + (d*g*m)/kr) + x4_hat*sin(x1_hat)*tan(x2_hat)) + (sin(x1_hat)*(x5_hat + (d*g*m)/kr) - x4_hat*cos(x1_hat))*(cos(x1_hat)*(x5_hat + (d*g*m)/kr)*(tan(x2_hat)^2 + 1) + x4_hat*sin(x1_hat)*(tan(x2_hat)^2 + 1)) + (sin(x1_hat)*tan(x2_hat)*(kr*x4_hat + x3_hat*(x5_hat + (d*g*m)/kr)*(Ixx - Izz)))/Ixx + (kr*x5_hat*cos(x1_hat)*tan(x2_hat))/Izz))/l - (2*Ixx*sin(x1_hat)*tan(x2_hat)*((cos(x1_hat)*(x5_hat + (d*g*m)/kr) + x4_hat*sin(x1_hat))*(x3_hat + cos(x1_hat)*tan(x2_hat)*(x5_hat + (d*g*m)/kr) + x4_hat*sin(x1_hat)*tan(x2_hat)) + (cos(x1_hat)*(kr*x4_hat + x3_hat*(x5_hat + (d*g*m)/kr)*(Ixx - Izz)))/Ixx - (kr*x5_hat*sin(x1_hat))/Izz))/(l*cos(x1_hat));
% alfa(2,1) = (kr*x5_hat*sin(x1_hat) - kr*x4_hat*cos(x1_hat) + d*g*m*sin(x1_hat))/cos(x1_hat) + (Ixx*((cos(x1_hat)*(kr*x4_hat + (x3_hat*(kr*x5_hat + d*g*m)*(Ixx - Izz))/kr))/Ixx + ((kr*x5_hat*cos(x1_hat) + kr*x4_hat*sin(x1_hat) + d*g*m*cos(x1_hat))*(x3_hat + x4_hat*sin(x1_hat)*tan(x2_hat) + (cos(x1_hat)*tan(x2_hat)*(kr*x5_hat + d*g*m))/kr))/kr - (kr*x5_hat*sin(x1_hat))/Izz))/cos(x1_hat) - (d*g*m*x1_hat)/cos(x1_hat) - (d*g*m*(2*Ixx - Izz)*(x3_hat + x4_hat*sin(x1_hat)*tan(x2_hat) + (cos(x1_hat)*tan(x2_hat)*(kr*x5_hat + d*g*m))/kr))/(kr*cos(x1_hat)) + (d^2*g^2*m^2*x2_hat*(Ixx - Izz))/(kr^2*cos(x1_hat));
% alfa(3,1) = 0;
% 
% beta = [
%         1, -(2*sin(x1_hat)*sin(x2_hat))/(l*cos(x1_hat)*cos(x2_hat)), -(2*Ixx*sin(x2_hat))/(Izz*l*cos(x1_hat)*cos(x2_hat));
%         0,                                            1/cos(x1_hat),                  (Ixx*sin(x1_hat))/(Izz*cos(x1_hat));
%         0,                                                        0,                                                    1];
    
u = alfa + beta*v;

== matlab function QuadCopter_3/LowLevelMotor/SaturationTr ==
  data: uf input; u output; d input; Tr input
function u = fcn(uf, d, Tr)

if abs(Tr) > d*uf
    Tr = sign(Tr)*d*uf;
end

u = Tr;

== matlab function QuadCopter_3/Inner Controller /Nonlinear Dynamics  ==
  data: x_hat_1 input; x_hat_2 input; x_hat_3 input; x_hat_4 input; x_hat_5 input; x_hat_dot output; u_hat input; constants input
function x_hat_dot = fcn(x_hat_1,x_hat_2,x_hat_3,x_hat_4,x_hat_5,u_hat,constants)

m= constants(1,1);
g= constants(2,1);
d= constants(3,1);
l= constants(4,1);
kr= constants(5,1);
Ixx= constants(6,1);
Iyy= constants(7,1);
Izz= constants(8,1);

x_hat = [x_hat_1;
        x_hat_2;
        x_hat_3;
        x_hat_4;
        x_hat_5];

f = [
    x_hat(3,1)+x_hat(4,1)*sin(x_hat(1,1))*tan(x_hat(2,1)) + ( x_hat(5,1)+ m*g*d/kr)*cos(x_hat(1,1))*tan(x_hat(2,1));
    x_hat(4,1)*cos(x_hat(1,1))- (x_hat(5,1)+ m*g*d/kr)*sin(x_hat(1,1)) ;
    1/Ixx*( -kr*x_hat(3,1)- x_hat(4,1)*(x_hat(5,1)+ m*g*d/kr)*(Izz - Ixx));
    1/Iyy*( -kr*x_hat(4,1)- x_hat(3,1)*(x_hat(5,1)+ m*g*d/kr)*(Ixx - Izz));
    1/Izz*(-kr* x_hat(5,1));    
    ];
G = [
    0 , 0 , 0;
    0,  0 , 0;
    l/(2*Ixx), 0 , -l/(2*d*Ixx)
    0,  1/Iyy  , 0 ;
    0 ,  0   ,  1/Izz;
    ];

    
x_hat_dot = f + G*u_hat;

== matlab function QuadCopter_3/LowLevelMotor/SaturationTq ==
  data: uf input; u output; d input; l input; Tr input; Tq input
function u = fcn(uf, d, l, Tr, Tq)

if abs(Tq) > (0.5*l*(uf+Tr/d))
    Tq = sign(Tq)*(0.5*l*(uf+Tr/d));
end

u = Tq;

== matlab function QuadCopter_3/ComputeInputs /boxMinus1 ==
  data: u2 input; diff output; u1 input
function diff = fcn(u2, u1)

R2 = [cos(u2) -sin(u2);
      sin(u2) cos(u2)];

R1 = [cos(-u1) -sin(-u1);
      sin(-u1) cos(-u1)];

R = R2*R1;

diff = atan2(R(2,1), R(1,1));

== matlab function QuadCopter_3/ComputeInputs /boxMinus2 ==
  data: u2 input; diff output; u1 input
function diff = fcn(u2, u1)

R2 = [cos(u2) -sin(u2);
      sin(u2) cos(u2)];

R1 = [cos(-u1) -sin(-u1);
      sin(-u1) cos(-u1)];

R = R2*R1;

diff = atan2(R(2,1), R(1,1));

== matlab function QuadCopter_3/Compute trajectory ==
  data: x_coeff input; pos output; y_coeff input; z_coeff input; t input; vel output; acc output
function [pos, vel, acc]  = fcn(x_coeff, y_coeff, z_coeff, t)

x = x_coeff(1)*t^3+x_coeff(2)*t^2+x_coeff(3)*t+x_coeff(4);
y = y_coeff(1)*t^3+y_coeff(2)*t^2+y_coeff(3)*t+y_coeff(4);
z = z_coeff(1)*t^3+z_coeff(2)*t^2+z_coeff(3)*t+z_coeff(4);

x_dot = 3*x_coeff(1)*t^2 +2*x_coeff(2)*t + x_coeff(3);
y_dot = 3*y_coeff(1)*t^2 +2*y_coeff(2)*t + y_coeff(3);
z_dot = 3*z_coeff(1)*t^2 +2*z_coeff(2)*t + z_coeff(3);

x_ddot = 6*x_coeff(1)*t+2*x_coeff(2);
y_ddot = 6*y_coeff(1)*t+2*y_coeff(2);
z_ddot = 6*z_coeff(1)*t+2*z_coeff(2);

u = zeros(3,1);

pos = [x, y, z]';
vel = [x_dot, y_dot, z_dot]';
acc = [x_ddot, y_ddot, z_ddot]';

== matlab function QuadCopter_3/Outer Controller /OuterControl ==
  data: psi input; x input; y input; z input; dx input; dy input; dz input; ddx input; ddy input; ddz input; phi_d output; pos input; vel input; acc input; theta_d output; r_d output; constants input
function [phi_d , theta_d , r_d ] = fcn(psi, x, y, z, dx, dy, dz, ddx, ddy, ddz, pos, vel, acc, constants)

m= constants(1,1);
g= constants(2,1);
d= constants(3,1);
l= constants(4,1);
kr= constants(5,1);
Ixx= constants(6,1);
Iyy= constants(7,1);
Izz= constants(8,1);
kt= constants(9,1);

xr = pos(1);
yr = pos(2);
zr = pos(3);

dxr = vel(1);
dyr = vel(2);
dzr = vel(3);

ddxr = acc(1);
ddyr = acc(2);
ddzr = acc(3);

R = [sin(psi), -cos(psi);
     cos(psi), sin(psi)];

% ux = kt/m*dx + ddxr + 0.008*(dxr -dx) + 0.03*(xr -x);
% uy = kt/m*dy + ddyr + 0.008*(dyr -dy) + 0.03*(yr -y);
% uz = kt/m*dz + ddzr + 0.5*(dzr -dz) + 0.15*(zr -z) + g;
ux = kt/m*dx + ddxr + 0.01*(dxr -dx) + 0.035*(xr -x);
uy = kt/m*dy + ddyr + 0.01*(dyr -dy) + 0.035*(yr -y);
uz = kt/m*dz + ddzr + 0.5*(dzr -dz) + 0.15*(zr -z) + g;

u = R*[ux, uy]';

r_d = uz*m*d/kr;
phi_d= u(2)/uz;
theta_d = u(1)/uz;

== matlab function QuadCopter_3/Nominal Quadrotor model/Quadrotor /MATLAB Function ==
  data: dx output; dy output; dz output; dx input; dy input; dz input; phi input; theta input; psi input; p input; q input; r input; uF input; ddx output; tauP input; tauQ input; tauR input; ddy output; ddz output; dp output; dq output; dr output; dphi output; dtheta output; dpsi output; constants input
function [dx,dy,dz,ddx,ddy,ddz,dp,dq,dr,dphi,dtheta,dpsi] = fcn(dx, dy, dz, phi, theta, psi, p, q, r, uF, tauP, tauQ, tauR, constants)

    m= constants(1,1);
    g= constants(2,1);
    d= constants(3,1);
    l= constants(4,1);
    kr= constants(5,1);
    Ixx= constants(6,1);
    Iyy= constants(7,1);
    Izz= constants(8,1);
    kt = constants(9,1);

    
    ddx = (1/m)*((cos(phi)*cos(psi)*sin(theta) + sin(phi)*sin(psi))*uF - kt*dx);
    
    ddy = (1/m)*((cos(phi)*sin(theta)*sin(psi) - cos(psi)*sin(phi))*uF - kt*dy);
    
    ddz = (1/m)*((cos(theta)*cos(phi))*uF - m*g - kt*dz);
    
%     dp = (1/Ixx)*(-kr*p - q*r*(Izz - Iyy) + tauP);

    dp = (1/Ixx)*(-kr*p - q*r*(Izz - Iyy) + l/2*(uF - tauR/d));
    
    dq = (1/Iyy)*(-kr*q - p*r*(Ixx - Izz) + tauQ);
    
    dr = (1/Izz)*(-kr*r - p*q*(Iyy - Ixx) + tauR);
    
%     dr = 1/Izz*(-kr*r + tauR);
    
    dphi = p + q*sin(phi)*tan(theta) + r*cos(phi)*tan(theta);
    
    dtheta = q*cos(phi) - r*sin(phi);
    
    dpsi = (1/cos(theta))*(q*sin(phi) + r*cos(phi));

== matlab function QuadCopter_3/Nominal Quadrotor model/Quadrotor /PeriodiZATOR ==
  data: u input; angle output
function angle = fcn(u)

y = sin(u);
x = cos(u);

% angle = mod(u, 2*pi)
angle = atan2(y,x);

== matlab function QuadCopter_3/Nominal Quadrotor model/Quadrotor /PeriodiZATOR1 ==
  data: u input; angle output
function angle = fcn(u)

y = sin(u);
x = cos(u);

% angle = mod(u, 2*pi)
angle = atan2(y,x);

== matlab function QuadCopter_3/Nominal Quadrotor model/Quadrotor /PeriodiZATOR2 ==
  data: u input; angle output
function angle = fcn(u)

y = sin(u);
x = cos(u);

% angle = mod(u, 2*pi);
angle = atan2(y,x);

== matlab function QuadCopter_3/Outer Controller /PeriodiZATOR3 ==
  data: u input; angle output
function angle = fcn(u)

y = sin(u);
x = cos(u);

% angle = mod(u, 2*pi);
angle = atan2(y,x);
